simulink model "plantModel_th"  (R2020a)
settings: Solver=VariableStepAuto  StartTime=0.0  StopTime=0.5  RelTol=1e-3
values from neighbouring files (symbols this model uses):
  csDef = [0;0;0]*pi/180    [AWE_Model_ts.m]    (also in plantModel_ts.m)
  G_vWind = [10;0;0]    [AWE_Model_ts.m]    (also in plantModel_ts.m = [0;0;0])
  thrDL = 0    [AWE_Model_ts.m]
  thrL = norm(init_G_rKite)    [AWE_Model_ts.m]    (also in plantModel_ts.m)
libraries: plantModel_cl x1
settings Model: Creator=Ayaz  LastModifiedBy=Ayaz

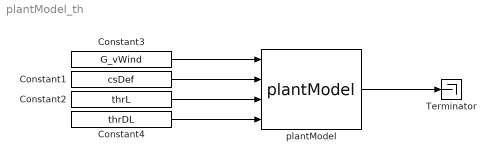
== system plantModel_th ==
  Constant1 : Constant  Value=csDef
  Constant2 : Constant  Value=thrL
  Constant3 : Constant  Value=G_vWind
  Constant4 : Constant  Value=thrDL
  Terminator : Terminator
  plantModel : plantModel_cl/plantModel  kiteMass=mass  kiteJmat=Jmat  refChord=refChord  refSpan=refSpan  refArea=refArea  xme_0=init_G_rKite  Vm_0=init_B_vKite  eul_0=init_Euler  pm_0=init_OwB  dThr=dTet  CdThr=rhoTet  thrSpringCns=TetKspring  rhoAir=rhoAir  gravAccl=gravAccl
  wires:
  Constant3/1 -> plantModel/1
  Constant1/1 -> plantModel/2
  plantModel/1 -> Terminator/1
  Constant2/1 -> plantModel/3
  Constant4/1 -> plantModel/4
